simulink model "asbhl20_FDIRmodelogicApp"  (R2016b)
settings: Solver=FixedStepDiscrete  StartTime=0.0  StopTime=65  FixedStep=Tf  RelTol=1e-3  AbsTol=1e-6  EnableMultiTasking=on
Description:
  | HL-20 FDIR reusable component for mode logic
settings Model: FPTRunName=Active  ModifiedByFormat=The MathWorks Inc.  SimulationMode=accelerator  Creator=The MathWorks, Inc.  LastModifiedBy=The MathWorks Inc.
settings DataIOCC: LimitDataPoints=on  SaveFormat=Array
settings OptimizationCC: DefaultParameterBehavior=Inlined  InlineInvariantSignals=on  ExpressionDepthLimit=2147483647  InitFltsAndDblsToZero=on  LifeSpan=1
settings DebuggingCC: SaveWithParameterizedLinksMsg=none  SolverPrmCheckMsg=warning  MultiTaskCondExecSysMsg=none  FcnCallInpInsideContextMsg=warning  UniqueDataStoreMsg=error  AllowSymbolicDim=off  StateNameClashWarn=warning  StrictBusMsg=ErrorOnBusTreatedAsVector  SFUnexpectedBacktrackingDiag=warning  SFNoUnconditionalDefaultTransitionDiag=warning  SFExecutionAtInitializationDiag=none
settings HardwareCC: ProdBitPerPointer=32  ProdBitPerSizeT=32  ProdBitPerPtrDiffT=32  ProdLargestAtomicFloat=None  ProdIntDivRoundTo=Undefined  ProdEndianess=Unspecified  ProdWordSize=32  ProdHWDeviceType=32-bit Generic
settings ModelReferenceCC: UpdateModelReferenceTargets=IfOutOfDate  PropagateSignalLabelsOutOfModel=off
settings SFSimCC: SimParseCustomCode=off
settings RTWCC: SystemTargetFile=ert.tlc  TemplateMakefile=ert_default_tmf  Description=RTW Embedded Coder (no auto configuration)
settings CodeAppCC: IgnoreCustomStorageClasses=off  CustomSymbolStrType=$N$R$M  InternalIdentifier=Classic
settings ERTTargetCC: TargetFcnLib=ansi_tfl_tmw.mat  GenerateSampleERTMain=on  SupportContinuousTime=on  SupportNonInlinedSFcns=on  InlinedParameterPlacement=NonHierarchical  ERTCustomFileTemplate=example_file_process.tlc  ConvertIfToSwitch=off  SuppressUnreachableDefaultCases=off
settings ConfigComp: CovMetricSettings=dw  CovHtmlReporting=on  CovSaveCumulativeToWorkspaceVar=on  CovSaveSingleToWorkspaceVar=on  CovExternalEMLEnable=off  CovSFcnEnable=off

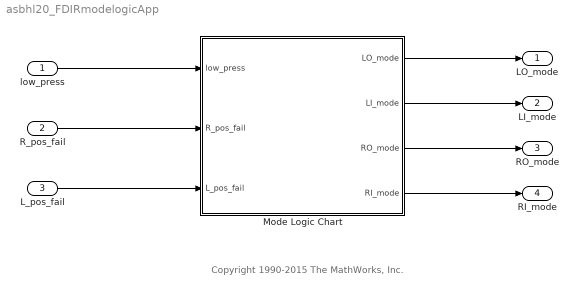
== system asbhl20_FDIRmodelogicApp ==
  note: Copyright 1990-2015 The MathWorks, Inc.
  low_press : Inport  OutDataTypeStr=boolean  PortDimensions=3
  R_pos_fail : Inport  Port=2  OutDataTypeStr=boolean  PortDimensions=2
  L_pos_fail : Inport  Port=3  OutDataTypeStr=boolean  PortDimensions=2
  Mode Logic Chart : Stateflow chart  TreatAsAtomicUnit=on
  LO_mode : Outport
  LI_mode : Outport  Port=2
  RO_mode : Outport  Port=3
  RI_mode : Outport  Port=4
  wires:
  low_press/1 -> Mode Logic Chart/1(low_press)
  R_pos_fail/1 -> Mode Logic Chart/2(R_pos_fail)
  L_pos_fail/1 -> Mode Logic Chart/3(L_pos_fail)
  Mode Logic Chart/1(LO_mode) -> LO_mode/1
  Mode Logic Chart/2(LI_mode) -> LI_mode/1
  Mode Logic Chart/3(RO_mode) -> RO_mode/1
  Mode Logic Chart/4(RI_mode) -> RI_mode/1

== stateflow chart asbhl20_FDIRmodelogicApp/Mode Logic Chart ==
  settings: sampleTime=0.5
  state Actuators
    en:L_switch();R_switch();
    du:L_switch();R_switch();
    state LO [parallel]
      settings: executionOrder=1
      state L1
        state passive
          LO_mode=2;
        state active
          LO_mode=4;
        state standby
          LO_mode=3;
        state off
          en:LO_mode=1;
          ex:fails++;
        (default) -> Actuators.LO.L1.passive
        Actuators.LO.L1.passive -> (junction 147) [order 2]
        (junction 147) -> Actuators.LO.L1.active : [!LI_act()|RO_act()]
        Actuators.LO.L1.standby -> (junction 147)
        Actuators.LO.L1.passive -> Actuators.LO.L1.standby [order 1] : [LI_act()]
        Actuators.LO.L1.active -> Actuators.LO.L1.standby : [!RO_act()&&...
            | LI_act()]
        Actuators.LO.L1 -> (junction 141) [order 1] : [off_LO && !in(off)]
        (junction 141) -> Actuators.LO.L1.off [order 2]
        Actuators.LO.L1.off -> Actuators.LO.L1 : [!low_press[1]]...
            | {off_LO=0;}
      state isolated
        LO_mode=0;
      (default) -> Actuators.LO.L1
      (junction 141) -> Actuators.LO.isolated [order 1] : [fails>=5]
      Actuators.LO.L1 -> Actuators.LO.isolated [order 1] : [isolated_LO]
    state RO [parallel]
      settings: executionOrder=2
      state L1
        state passive
          RO_mode=2;
        state active
          RO_mode=4;
        state standby
          RO_mode=3;
        state off
          en:RO_mode=1;
          ex:fails++;
        (default) -> Actuators.RO.L1.passive
        Actuators.RO.L1.passive -> (junction 154) [order 2]
        (junction 154) -> Actuators.RO.L1.active : [!RI_act()|LO_act()]
        Actuators.RO.L1.standby -> (junction 154)
        Actuators.RO.L1.passive -> Actuators.RO.L1.standby [order 1] : [RI_act()]
        Actuators.RO.L1.active -> Actuators.RO.L1.standby : [!LO_act()&&...
            | RI_act()]
        Actuators.RO.L1.off -> Actuators.RO.L1 : [!low_press[3]]...
            | {off_RO=0;}
        Actuators.RO.L1 -> (junction 153) [order 1] : [off_RO && !in(off)]
        (junction 153) -> Actuators.RO.L1.off [order 2]
      state isolated
        RO_mode=0;
      (default) -> Actuators.RO.L1
      (junction 153) -> Actuators.RO.isolated [order 1] : [fails>=5]
      Actuators.RO.L1 -> Actuators.RO.isolated [order 1] : [isolated_RO]
    state LI [parallel]
      settings: executionOrder=3
      state L1
        state passive
          LI_mode=2;
        state active
          LI_mode=4;
        state standby
          LI_mode=3;
        state off
          en:LI_mode=1;
          ex:fails++;
        (default) -> Actuators.LI.L1.passive
        Actuators.LI.L1.passive -> (junction 152) [order 2]
        (junction 152) -> Actuators.LI.L1.active : [!LO_act()|RI_act()]
        Actuators.LI.L1.standby -> (junction 152)
        Actuators.LI.L1.passive -> Actuators.LI.L1.standby [order 1] : [LO_act()]
        Actuators.LI.L1.active -> Actuators.LI.L1.standby : [RO_act()&&...
            | LO_act()]
        Actuators.LI.L1.off -> Actuators.LI.L1 : [!low_press[2]]...
            | {off_LI=0;}
        Actuators.LI.L1 -> (junction 151) [order 1] : [off_LI && !in(off)]
        (junction 151) -> Actuators.LI.L1.off [order 2]
      state isolated
        LI_mode=0;
      (default) -> Actuators.LI.L1
      (junction 151) -> Actuators.LI.isolated [order 1] : [fails>=5]
      Actuators.LI.L1 -> Actuators.LI.isolated [order 1] : [isolated_LI]
    state RI [parallel]
      settings: executionOrder=4
      state L1
        state passive
          RI_mode=2;
        state active
          RI_mode=4;
        state standby
          RI_mode=3;
        state off
          en:RI_mode=1;
          ex:fails++;
        (default) -> Actuators.RI.L1.passive
        Actuators.RI.L1.passive -> (junction 150) [order 2]
        (junction 150) -> Actuators.RI.L1.active : [!RO_act()|LI_act()]
        Actuators.RI.L1.standby -> (junction 150)
        Actuators.RI.L1.passive -> Actuators.RI.L1.standby [order 1] : [RO_act()]
        Actuators.RI.L1.active -> Actuators.RI.L1.standby : [LO_act()&&...
            | RO_act()]
        Actuators.RI.L1 -> (junction 149) [order 1] : [off_RI && in(off)]
        (junction 149) -> Actuators.RI.L1.off [order 2]
        Actuators.RI.L1.off -> Actuators.RI.L1 : [!low_press[2]]...
            | {off_RI=0;}
      state isolated
        RI_mode=0;
      (default) -> Actuators.RI.L1
      (junction 149) -> Actuators.RI.isolated [order 1] : [fails>=5]
      Actuators.RI.L1 -> Actuators.RI.isolated [order 1] : [isolated_RI]
  state L_switch [function]
    (default) -> (junction 247)
    (junction 247) -> (junction 249) : {
        | /* Hydraulic system 1 Low pressure (Left Outer line) */
        | aVarTruthTableCondition_1 = (low_press[1]);
        | }
    (junction 249) -> (junction 251) : {
        | /* Left Outer actuator position failed */
        | aVarTruthTableCondition_2 = (L_pos_fail[1]);
        | }
    (junction 251) -> (junction 253) : {
        | /* Hydraulic system 2 Low pressure (Inner line) */
        | aVarTruthTableCondition_3 = (low_press[2]);
        | }
    (junction 253) -> (junction 255) : {
        | /* Left Inner actuator position failed */
        | aVarTruthTableCondition_4 = (L_pos_fail[2]);
        | }
    (junction 255) -> (junction 257) [order 1] : [aVarTruthTableCondition_1 && !aVarTruthTableCondition_3 && !aVarTruthTableCondition_4]
    (junction 257) -> (junction 259) : {
        | /* Hydraulic System 1 Failure. Turn off Left Outer Actuator */
        | off_LO=1;
        | }
    (junction 255) -> (junction 261) [order 2]
    (junction 261) -> (junction 263) [order 1] : [aVarTruthTableCondition_1]
    (junction 263) -> (junction 265) : {
        | /* Left Outer Actuator Failure. Isolate Left Outer Actuator */
        | isolated_LO=1;
        | }
    (junction 265) -> (junction 267) : {
        | /* Left Inner Actuator Failure. Isolate Left Inner Actuator */
        | isolated_LI=1;
        | }
    (junction 261) -> (junction 269) [order 2]
    (junction 269) -> (junction 271) [order 1] : [!aVarTruthTableCondition_1 && aVarTruthTableCondition_2 && !aVarTruthTableCondition_3 && !aVarTruthTableCondition_4]
    (junction 271) -> (junction 273) : {
        | /* Left Outer Actuator Failure. Isolate Left Outer Actuator */
        | isolated_LO=1;
        | }
    (junction 269) -> (junction 275) [order 2]
    (junction 275) -> (junction 277) [order 1] : [!aVarTruthTableCondition_1 && aVarTruthTableCondition_2]
    (junction 277) -> (junction 279) : {
        | /* Left Outer Actuator Failure. Isolate Left Outer Actuator */
        | isolated_LO=1;
        | }
    (junction 279) -> (junction 281) : {
        | /* Left Inner Actuator Failure. Isolate Left Inner Actuator */
        | isolated_LI=1;
        | }
    (junction 275) -> (junction 283) [order 2]
    (junction 283) -> (junction 285) [order 1] : [aVarTruthTableCondition_3]
    (junction 285) -> (junction 287) : {
        | /* Hydraulic System 2 Failure. Turn off Left Inner Actuator */
        | off_LI=1;
        | }
    (junction 283) -> (junction 289) [order 2]
    (junction 289) -> (junction 291) [order 1] : [aVarTruthTableCondition_4]
    (junction 291) -> (junction 293) : {
        | /* Left Inner Actuator Failure. Isolate Left Inner Actuator */
        | isolated_LI=1;
        | }
    (junction 289) -> (junction 295) [order 2]
    (junction 295) -> (junction 297) : /* Default */
    (junction 297) -> (junction 299) : {
        | /* 'Default':Default - All ok, do nothing. */
        |
        | }
  state R_switch [function]
    (default) -> (junction 305)
    (junction 305) -> (junction 307) : {
        | /* Hydraulic system 3 Low pressure (Right Outer line) */
        | aVarTruthTableCondition_1 = (low_press[3]);
        | }
    (junction 307) -> (junction 309) : {
        | /* Right Outer actuator position failed */
        | aVarTruthTableCondition_2 = (R_pos_fail[1]);
        | }
    (junction 309) -> (junction 311) : {
        | /* Hydraulic system 2 Low pressure (Inner line) */
        | aVarTruthTableCondition_3 = (low_press[2]);
        | }
    (junction 311) -> (junction 313) : {
        | /* Right Inner actuator position failed */
        | aVarTruthTableCondition_4 = (R_pos_fail[2]);
        | }
    (junction 313) -> (junction 315) [order 1] : [aVarTruthTableCondition_1 && !aVarTruthTableCondition_3 && !aVarTruthTableCondition_4]
    (junction 315) -> (junction 317) : {
        | /* Hydraulic System 3 Failure. Turn off Right Outer Actuator */
        | off_RO=1;
        | }
    (junction 313) -> (junction 319) [order 2]
    (junction 319) -> (junction 321) [order 1] : [aVarTruthTableCondition_1]
    (junction 321) -> (junction 323) : {
        | /* Mulitple Failure. Isolate Right Outer AND Right Inner Actuators */
        | isolated_RO=1;
        | isolated_RI=1;
        | }
    (junction 319) -> (junction 325) [order 2]
    (junction 325) -> (junction 327) [order 1] : [!aVarTruthTableCondition_1 && aVarTruthTableCondition_2 && !aVarTruthTableCondition_3 && !aVarTruthTableCondition_4]
    (junction 327) -> (junction 329) : {
        | /* Right Outer Actuator Failure. Isolate Right Outer Actuator */
        | isolated_RO=1;
        | }
    (junction 325) -> (junction 331) [order 2]
    (junction 331) -> (junction 333) [order 1] : [!aVarTruthTableCondition_1 && aVarTruthTableCondition_2]
    (junction 333) -> (junction 335) : {
        | /* Mulitple Failure. Isolate Right Outer AND Right Inner Actuators */
        | isolated_RO=1;
        | isolated_RI=1;
        | }
    (junction 331) -> (junction 337) [order 2]
    (junction 337) -> (junction 339) [order 1] : [aVarTruthTableCondition_3]
    (junction 339) -> (junction 341) : {
        | /* Hydraulic System 2 Failure. Turn off Right Inner Actuator */
        | off_RI=1;
        | }
    (junction 337) -> (junction 343) [order 2]
    (junction 343) -> (junction 345) [order 1] : [aVarTruthTableCondition_4]
    (junction 345) -> (junction 347) : {
        | /* Right Inner Actuator Failure. Isolate Right Inner Actuator */
        | isolated_RI=1;
        | }
    (junction 343) -> (junction 349) [order 2]
    (junction 349) -> (junction 351) : /* Default */
    (junction 351) -> (junction 353) : {
        | /* 'Default':Default - All ok, do nothing. */
        |
        | }
  state y = LI_act [function]
    (default) -> (junction 160) : {y=in(Actuators.LI.L1.active);}
  state y = RO_act [function]
    (default) -> (junction 158) : {y=in(Actuators.RO.L1.active);}
  state y = LO_act [function]
    (default) -> (junction 159) : {y=in(Actuators.LO.L1.active);}
  state y = RI_act [function]
    (default) -> (junction 157) : {y=in(Actuators.RI.L1.active);}
  note: This mode logic assumes that there are 3 hydraulic lines, one that is connected to the 2 redundant actuators (Left Inner and Right Inner actuators).
      | The other two are connected to the primary actuators Left Outer and Right Outer (1 per actuator).
  data: fails local int32; fails local int32; fails local int32; fails local int32; aVarTruthTableCondition_1 temporary boolean =0; aVarTruthTableCondition_2 temporary boolean =0; aVarTruthTableCondition_3 temporary boolean =0; aVarTruthTableCondition_4 temporary boolean =0; aVarTruthTableCondition_1 temporary boolean =0; aVarTruthTableCondition_2 temporary boolean =0; aVarTruthTableCondition_3 temporary boolean =0; aVarTruthTableCondition_4 temporary boolean =0; y function_output double; y function_output double; y function_output double; y function_output double; low_press input boolean size=3; LO_mode output int8 size=1 [0..4]; LI_mode output int8 size=1 [0..4]; R_pos_fail input boolean size=2; L_pos_fail input boolean size=2; RO_mode output int8 size=1 [0..4]; RI_mode output int8 size=1 [0..4]; isolated_LI local double; isolated_LO local double; isolated_RI local double; isolated_RO local double; off_LI local double; off_LO local double; off_RI local double; off_RO local double
  data aVarTruthTableCondition_1 settings: description=Hydraulic system 1 Low pressure (Left Outer line)
  data aVarTruthTableCondition_2 settings: description=Left Outer actuator position failed
  data aVarTruthTableCondition_3 settings: description=Hydraulic system 2 Low pressure (Inner line)
  data aVarTruthTableCondition_4 settings: description=Left Inner actuator position failed
  data aVarTruthTableCondition_1 settings: description=Hydraulic system 3 Low pressure (Right Outer line)
  data aVarTruthTableCondition_2 settings: description=Right Outer actuator position failed
  data aVarTruthTableCondition_3 settings: description=Hydraulic system 2 Low pressure (Inner line)
  data aVarTruthTableCondition_4 settings: description=Right Inner actuator position failed
